simulink subsystem "getGyroData"  (R2024a)
settings: Solver=VariableStepAuto  StartTime=0.0  StopTime=10.0  RelTol=1e-3
undefined symbols (not defined in the file or in its folder): angleEstRate, bits
libraries: stm32blockslib x12
settings Model: Creator=Peter  LastModifiedBy=Peter

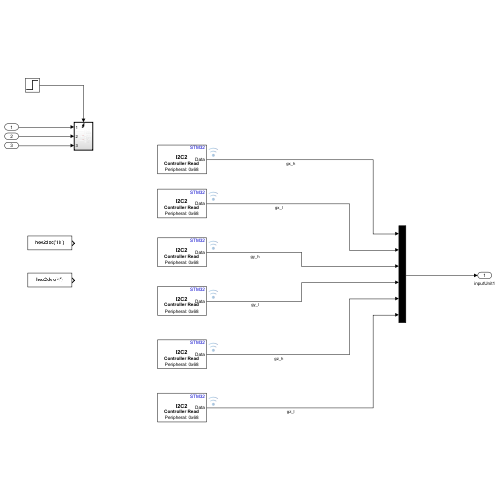
[thumbnail: Simulink's stored preview of the top-level diagram]
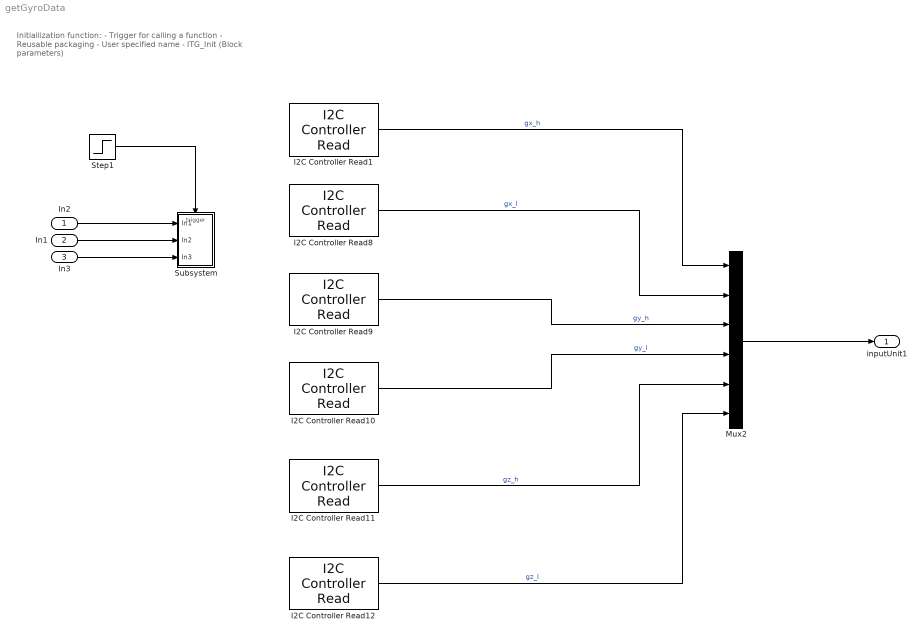
== system getGyroData ==
  note: Initiallization function:
      | - Trigger for calling a function
      | - Reusable packaging
      | - User specified name
      | - ITG_Init (Block parameters)
  In2 : Inport
  In1 : Inport  Port=2
  In3 : Inport  Port=3
  I2C Controller Read1 : stm32blockslib/I2C Controller Read  I2CModule=I2C2  Mode=Controller  AddressingMode=7-bits  PeripheralByteOrder=LittleEndian  OwnPeripheralAddress=uint8(170)  PeripheralAddressVia=Dialog  PeripheralAddress=hex2dec('68')  RegisterAddressMode=on  RegisterAddressVia=Dialog  RegisterAddress=uint8(hex2dec('1D'))  RepeatedStart=off  NoAck=off  OutputStatus=off  BlockMode=Receive  DataType=uint8  DataLength=1  Timeout=0.001  SampleTime=angleEstRate
      settings: LibrarySourceBlock=stm32f7xxblockslib/I2C Controller Read
  I2C Controller Read10 : stm32blockslib/I2C Controller Read  I2CModule=I2C2  Mode=Controller  AddressingMode=7-bits  PeripheralByteOrder=LittleEndian  OwnPeripheralAddress=uint8(170)  PeripheralAddressVia=Dialog  PeripheralAddress=hex2dec('68')  RegisterAddressMode=on  RegisterAddressVia=Dialog  RegisterAddress=uint8(hex2dec('20'))  RepeatedStart=off  NoAck=off  OutputStatus=off  BlockMode=Receive  DataType=uint8  DataLength=1  Timeout=0.001  SampleTime=angleEstRate
      settings: LibrarySourceBlock=stm32f7xxblockslib/I2C Controller Read
  I2C Controller Read11 : stm32blockslib/I2C Controller Read  I2CModule=I2C2  Mode=Controller  AddressingMode=7-bits  PeripheralByteOrder=LittleEndian  OwnPeripheralAddress=uint8(170)  PeripheralAddressVia=Dialog  PeripheralAddress=hex2dec('68')  RegisterAddressMode=on  RegisterAddressVia=Dialog  RegisterAddress=uint8(hex2dec('21'))  RepeatedStart=off  NoAck=off  OutputStatus=off  BlockMode=Receive  DataType=uint8  DataLength=1  Timeout=0.001  SampleTime=angleEstRate
      settings: LibrarySourceBlock=stm32f7xxblockslib/I2C Controller Read
  I2C Controller Read12 : stm32blockslib/I2C Controller Read  I2CModule=I2C2  Mode=Controller  AddressingMode=7-bits  PeripheralByteOrder=LittleEndian  OwnPeripheralAddress=uint8(170)  PeripheralAddressVia=Dialog  PeripheralAddress=hex2dec('68')  RegisterAddressMode=on  RegisterAddressVia=Dialog  RegisterAddress=uint8(hex2dec('22'))  RepeatedStart=off  NoAck=off  OutputStatus=off  BlockMode=Receive  DataType=uint8  DataLength=1  Timeout=0.001  SampleTime=angleEstRate
      settings: LibrarySourceBlock=stm32f7xxblockslib/I2C Controller Read
  I2C Controller Read8 : stm32blockslib/I2C Controller Read  I2CModule=I2C2  Mode=Controller  AddressingMode=7-bits  PeripheralByteOrder=LittleEndian  OwnPeripheralAddress=uint8(170)  PeripheralAddressVia=Dialog  PeripheralAddress=hex2dec('68')  RegisterAddressMode=on  RegisterAddressVia=Dialog  RegisterAddress=uint8(hex2dec('1E'))  RepeatedStart=off  NoAck=off  OutputStatus=off  BlockMode=Receive  DataType=uint8  DataLength=1  Timeout=0.001  SampleTime=angleEstRate
      settings: LibrarySourceBlock=stm32f7xxblockslib/I2C Controller Read
  I2C Controller Read9 : stm32blockslib/I2C Controller Read  I2CModule=I2C2  Mode=Controller  AddressingMode=7-bits  PeripheralByteOrder=LittleEndian  OwnPeripheralAddress=uint8(170)  PeripheralAddressVia=Dialog  PeripheralAddress=hex2dec('68')  RegisterAddressMode=on  RegisterAddressVia=Dialog  RegisterAddress=uint8(hex2dec('1F'))  RepeatedStart=off  NoAck=off  OutputStatus=off  BlockMode=Receive  DataType=uint8  DataLength=1  Timeout=0.001  SampleTime=angleEstRate
      settings: LibrarySourceBlock=stm32f7xxblockslib/I2C Controller Read
  Mux2 : Mux  Inputs=6
  Step1 : Step
  Subsystem : Subsystem  RTWFcnName=ITG_Init
      settings: RTWFcnNameOpts=User specified
  inputUnit1 : Outport  VectorParamsAs1DForOutWhenUnconnected=off
  wires:
  I2C Controller Read1/1 -> Mux2/1  "gx_h"
  I2C Controller Read9/1 -> Mux2/3  "gy_h"
  Step1/1 -> Subsystem/Trigger
  I2C Controller Read11/1 -> Mux2/5  "gz_h"
  Mux2/1 -> inputUnit1/1
  I2C Controller Read12/1 -> Mux2/6  "gz_l"
  I2C Controller Read8/1 -> Mux2/2  "gx_l"
  In2/1 -> Subsystem/1(In1)
  I2C Controller Read10/1 -> Mux2/4  "gy_l"
  In1/1 -> Subsystem/2(In2)
  In3/1 -> Subsystem/3(In3)

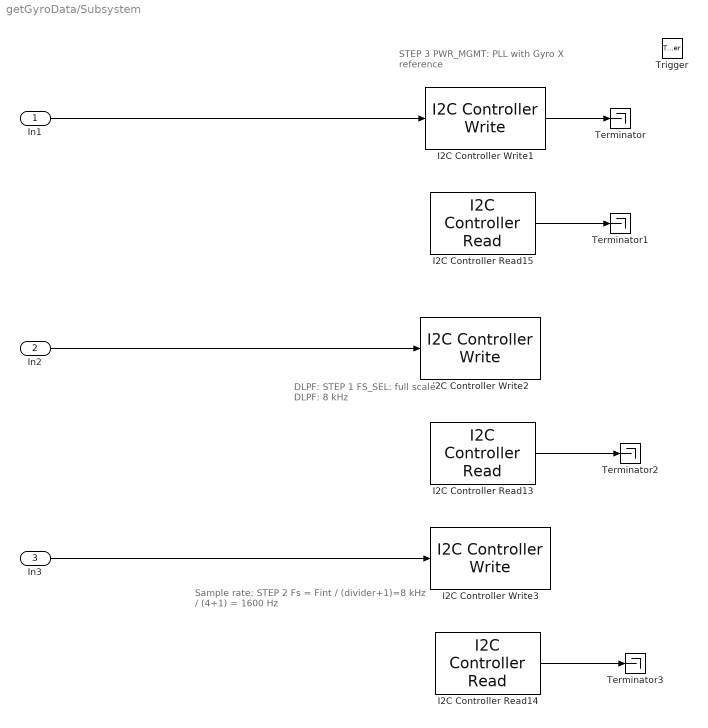
== system getGyroData/Subsystem ==
  note: STEP 3
      | PWR_MGMT: PLL with Gyro X reference
  note: Sample rate: STEP 2
      | Fs = Fint / (divider+1)=8 kHz / (4+1) = 1600 Hz
  note: DLPF: STEP 1
      | FS_SEL: full scale
      | DLPF: 8 kHz
  In1 : Inport
  In2 : Inport  Port=2
  In3 : Inport  Port=3
  Trigger : TriggerPort  VariantControl=(inherit)  PortDimensions=1
  I2C Controller Read13 : stm32blockslib/I2C Controller Read  Priority=-5  I2CModule=I2C2  Mode=Controller  AddressingMode=7-bits  PeripheralByteOrder=LittleEndian  OwnPeripheralAddress=uint8(170)  PeripheralAddressVia=Dialog  PeripheralAddress=hex2dec('68')  RegisterAddressMode=on  RegisterAddressVia=Dialog  RegisterAddress=uint8(hex2dec('16'))  RepeatedStart=off  NoAck=off  OutputStatus=off  BlockMode=Receive  DataType=uint8  DataLength=1  Timeout=0.001  SampleTime=inf
      settings: LibrarySourceBlock=stm32f7xxblockslib/I2C Controller Read
  I2C Controller Read14 : stm32blockslib/I2C Controller Read  Priority=-3  I2CModule=I2C2  Mode=Controller  AddressingMode=7-bits  PeripheralByteOrder=LittleEndian  OwnPeripheralAddress=uint8(170)  PeripheralAddressVia=Dialog  PeripheralAddress=hex2dec('68')  RegisterAddressMode=on  RegisterAddressVia=Dialog  RegisterAddress=uint8(hex2dec('15'))  RepeatedStart=off  NoAck=off  OutputStatus=off  BlockMode=Receive  DataType=uint8  DataLength=1  Timeout=0.001  SampleTime=inf
      settings: LibrarySourceBlock=stm32f7xxblockslib/I2C Controller Read
  I2C Controller Read15 : stm32blockslib/I2C Controller Read  Priority=-1  I2CModule=I2C2  Mode=Controller  AddressingMode=7-bits  PeripheralByteOrder=LittleEndian  OwnPeripheralAddress=uint8(170)  PeripheralAddressVia=Dialog  PeripheralAddress=hex2dec('68')  RegisterAddressMode=on  RegisterAddressVia=Dialog  RegisterAddress=uint8(hex2dec('3E'))  RepeatedStart=off  NoAck=off  OutputStatus=off  BlockMode=Receive  DataType=uint8  DataLength=1  Timeout=0.001  SampleTime=inf
      settings: LibrarySourceBlock=stm32f7xxblockslib/I2C Controller Read
  I2C Controller Write1 : stm32blockslib/I2C Controller Write  Priority=-2  I2CModule=I2C2  Mode=Controller  AddressingMode=7-bits  PeripheralByteOrder=LittleEndian  OwnPeripheralAddress=uint8(170)  PeripheralAddressVia=Dialog  PeripheralAddress=hex2dec('68')  RegisterAddressMode=on  RegisterAddressVia=Dialog  RegisterAddress=uint8(hex2dec('3E'))  RepeatedStart=off  NoAck=off  OutputStatus=on  BlockMode=Transmit  DataType=uint8  DataLength=1  Timeout=0.001  SampleTime=-1
      settings: LibrarySourceBlock=stm32f7xxblockslib/I2C Controller Write
  I2C Controller Write2 : stm32blockslib/I2C Controller Write  Priority=-6  I2CModule=I2C2  Mode=Controller  AddressingMode=7-bits  PeripheralByteOrder=LittleEndian  OwnPeripheralAddress=uint8(170)  PeripheralAddressVia=Dialog  PeripheralAddress=hex2dec('68')  RegisterAddressMode=on  RegisterAddressVia=Dialog  RegisterAddress=uint8(hex2dec('16'))  RepeatedStart=off  NoAck=off  OutputStatus=off  BlockMode=Transmit  DataType=uint8  DataLength=1  Timeout=0.001  SampleTime=-1
      settings: LibrarySourceBlock=stm32f7xxblockslib/I2C Controller Write
  I2C Controller Write3 : stm32blockslib/I2C Controller Write  Priority=-4  I2CModule=I2C2  Mode=Controller  AddressingMode=7-bits  PeripheralByteOrder=LittleEndian  OwnPeripheralAddress=uint8(170)  PeripheralAddressVia=Dialog  PeripheralAddress=hex2dec('68')  RegisterAddressMode=on  RegisterAddressVia=Dialog  RegisterAddress=uint8(hex2dec('15'))  RepeatedStart=off  NoAck=off  OutputStatus=off  BlockMode=Transmit  DataType=uint8  DataLength=1  Timeout=0.001  SampleTime=-1
      settings: LibrarySourceBlock=stm32f7xxblockslib/I2C Controller Write
  Terminator{,1..3} (4 alike) : Terminator
  wires:
  I2C Controller Write1/1 -> Terminator/1
  I2C Controller Read14/1 -> Terminator3/1
  I2C Controller Read13/1 -> Terminator2/1
  In2/1 -> I2C Controller Write2/1
  In1/1 -> I2C Controller Write1/1
  I2C Controller Read15/1 -> Terminator1/1
  In3/1 -> I2C Controller Write3/1
